simulink model "mech_stewart_control"  (Simulink 6.0)
settings: Solver=ode45  StartTime=0.0  StopTime=10.0  RelTol=1e-3
PreLoadFcn:
  | mech_stewart_control_setup
PostLoadFcn:
  | find_system(gcs,'FollowLinks', 'on', 'LookUnderMasks', 'all');set_param(gcs,'SimulationCommand','update');
undefined symbols (not defined in the file or in its folder): body_pts, pos_base, top_inertia, top_mass
libraries: simulink x10, mblibv1 x9, mech_stewartplatform_leg x6, mech_stewart_controllers x1, mech_stewart_control_deriv x1
Description:
  | Stewart platform controls case study: complete control system with
  | controller and plant.
  | 
  | Controller is one of the enabled subsystems of:
  | toolbox/physmod/mech/mechdemos/mech_stewart_controllers.mdl.
  | 
  | Plant subsystem uses leg instances of the linked library:
  | toolbox/physmod/mech/mechdemos/mech_stewartplatform_leg.mdl.
settings Model: Creator=dkennedy  LastModifiedBy=batserve  ExtModeAutoUpdateStatusClock=off
settings DataIOCC: SignalLoggingName=sigsOut  OutputTimes=[0:0.01:50]
settings OptimizationCC: BooleanDataType=off
settings DebuggingCC: CheckExecutionContextPreStartOutputMsg=on  CheckExecutionContextRuntimeOutputMsg=on  SolverPrmCheckMsg=none
settings HardwareCC: TargetUnknown=on
settings CodeAppCC: MangleLength=5
settings SimMechanicsCC: VisOnUpdateDiagram=on  VisDuringSimulation=on

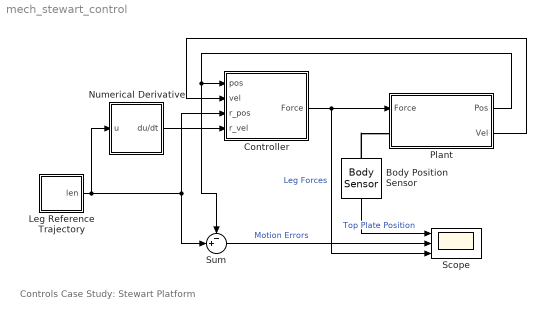
== system mech_stewart_control ==
  note: Controls Case Study:
      | Stewart Platform
  Body Position Sensor : mblibv1/Sensors &  Actuators/Body Sensor  Orientation=down  Opaque=on  PhysicalDomain=Mechanical  PortType=blob  Muxed=on  Pose=off  Angle=on  AngleUnits=deg  ArcVelocity=off  ArcVelocityUnits=deg/s  ArcAcceleration=off  ArcAccelerationUnits=deg/s^2  CoordPosition=on  CoordPositionUnits=m  Velocity=off  VelocityUnits=m/s  Acceleration=off  AccelerationUnits=m/s^2  Quaternion=on  QuaternionDT=off  QuaternionDDT=off  QuaternionUnits=off  OutputVector=[ 3 ]  ActiveIO=on  Width=3  DialogClass=MechanicalSensorBlock  ReferenceFrame=Absolute (World)
  "Controller " : Subsystem  BlockChoice=Null Controller
      settings: AttributesFormatString=%<BlockChoice>  TemplateBlock=mech_stewart_controllers/Controller  MemberBlocks=H_inf Controller,Null Controller,PID Controller
  Leg Reference Trajectory : Subsystem
  "Numerical Derivative " : Subsystem  BlockChoice=Derivative Block
      settings: AttributesFormatString=%<BlockChoice>  MemberBlocks=Derivative Block,Filtered Derivative
      settings: TemplateBlock=|
      | mech_stewart_control_deriv/Numerical
      | Derivative
  Plant : Subsystem
  Scope : Scope  NumInputPorts=3
      settings: Tag=OpenMeAtStartUp  TimeRange=1  YMin=-3~-1~-1  YMax=2~3~1
  Sum : Sum  Inputs=-+|  SaturateOnIntegerOverflow=on  InputSameDT=on
  wires:
  Plant/1(Pos) -> Sum/1, "Controller "/1(pos)
  "Controller "/1(Force) -> Plant/1(Force), Scope/3  "Leg Forces"
  Sum/1 -> Scope/2  "Motion Errors"
  Leg Reference Trajectory/1(len) -> "Numerical Derivative "/1(u), Sum/2, "Controller "/3(r_pos)
  Body Position Sensor/1 -> Scope/1  "Top Plate Position"
  Plant/2(Vel) -> "Controller "/2(vel)
  "Numerical Derivative "/1(du/dt) -> "Controller "/4(r_vel)
  connections:
  Body Position Sensor/LConn1 -- Plant/LConn1

== system mech_stewart_control/Controller  ==
  pos : Inport  Port=1  LatchInput=off
  vel : Inport  Port=2  LatchInput=off
  r_pos : Inport  Port=3  LatchInput=off
  r_vel : Inport  Port=4  LatchInput=off
  Null Controller : mech_stewart_controllers/Null Controller
  Force : Outport
  wires:
  pos/1 -> Null Controller/1
  vel/1 -> Null Controller/2
  r_pos/1 -> Null Controller/3
  r_vel/1 -> Null Controller/4
  Null Controller/1 -> Force/1

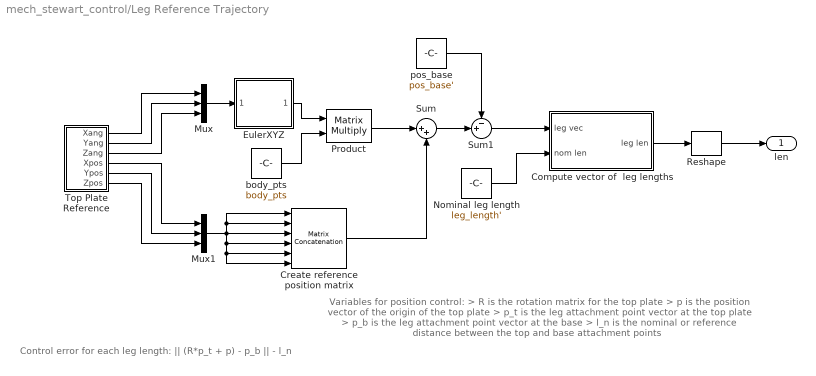
== system mech_stewart_control/Leg Reference Trajectory ==
  note: Variables for position control:
      |
      | > R is the rotation matrix  for the top plate
      | > p is the position vector of the origin of the top plate
      | > p_t is the leg attachment point vector at the top plate
      | > p_b is the leg attachment point vector at the base
      | > l_n is the nominal or reference distance between the
      |    top and base attachment points
  note: Control error for each leg length:
      |
      |    || (R*p_t + p) - p_b || - l_n
  Compute vector of  leg lengths : Subsystem  TreatAsAtomicUnit=on
  Create reference position matrix : simulink/Math Operations/Matrix Concatenation  numInports=6  catMethod=Horizontal
  EulerXYZ : Subsystem  AncestorBlock=|
      | aerospace/Axes
      | Transformations/Direction Cosine Matrix
      | from Euler Angles
      mask Type: EulerXYZ
      mask Description: Creates the EulerXYZ rotation matrix corresponding to body fixed rotations in the X, Y, and then Z. This matrix maps body vectors to world vectors.
      mask Help:
      | <p>This block determines the EulerXYZ matrix from a 3x1 euler angles in the X, Y, & Z directions. The matrix maps vectors the body axes to the inertial axes.</p>
      | 
      | <p>The block input and output contain more than one signal as described below.</p>
      | 
      | <p><H4>Block Vector Input - Euler XYZ angles</H4>
      |     <ul>
      |     <li>X angle</li>
      |     <li>Y angle</li>
      |     <li>Z angle</li>
      |    </ul>
      |    </p>
      | 
      | <p><H4>Block Matrix Output - XYZ Euler Matrix </H4>
      |     <ul>
      |    </ul>
      |    </p>
      mask Display: disp('Rotation\nMatrix')
  Mux : Mux  Inputs=3
  Mux1 : Mux  Inputs=3
  Nominal leg length : Constant  Value=leg_length'  VectorParams1D=off
  Product : Product  Multiplication=Matrix(*)  SaturateOnIntegerOverflow=on  InputSameDT=on
  Reshape : simulink/Math Operations/Reshape  OutputDimensionality=1-D array  OutputDimensions=[1,1]
  Sum : Sum  Inputs=|++  SaturateOnIntegerOverflow=on  InputSameDT=on
  Sum1 : Sum  Inputs=-+|  SaturateOnIntegerOverflow=on  InputSameDT=on
  Top Plate Reference : Subsystem
  body_pts : Constant  Value=body_pts  VectorParams1D=off
  pos_base : Constant  Value=pos_base'  VectorParams1D=off
  len : Outport
  wires:
  Mux/1 -> EulerXYZ/1(x y z angles)
  EulerXYZ/1(EulerXYZ) -> Product/1
  body_pts/1 -> Product/2
  Product/1 -> Sum/1
  Mux1/1 -> Create reference position matrix/3, Create reference position matrix/1, Create reference position matrix/2, Create reference position matrix/4, Create reference position matrix/5, Create reference position matrix/6
  Create reference position matrix/1 -> Sum/2
  pos_base/1 -> Sum1/1
  Sum/1 -> Sum1/2
  Sum1/1 -> Compute vector of  leg lengths/1(leg vec)
  Nominal leg length/1 -> Compute vector of  leg lengths/2(nom len)
  Compute vector of  leg lengths/1(leg len) -> Reshape/1
  Top Plate Reference/3(Zang) -> Mux/3
  Top Plate Reference/1(Xang) -> Mux/1
  Top Plate Reference/2(Yang) -> Mux/2
  Top Plate Reference/4(Xpos) -> Mux1/1
  Top Plate Reference/5(Ypos) -> Mux1/2
  Top Plate Reference/6(Zpos) -> Mux1/3
  Reshape/1 -> len/1

== system mech_stewart_control/Numerical Derivative  ==
  u : Inport  Port=1  LatchInput=off
  Derivative Block : mech_stewart_control_deriv/Derivative Block
  du/dt : Outport
  wires:
  u/1 -> Derivative Block/1
  Derivative Block/1 -> du/dt/1

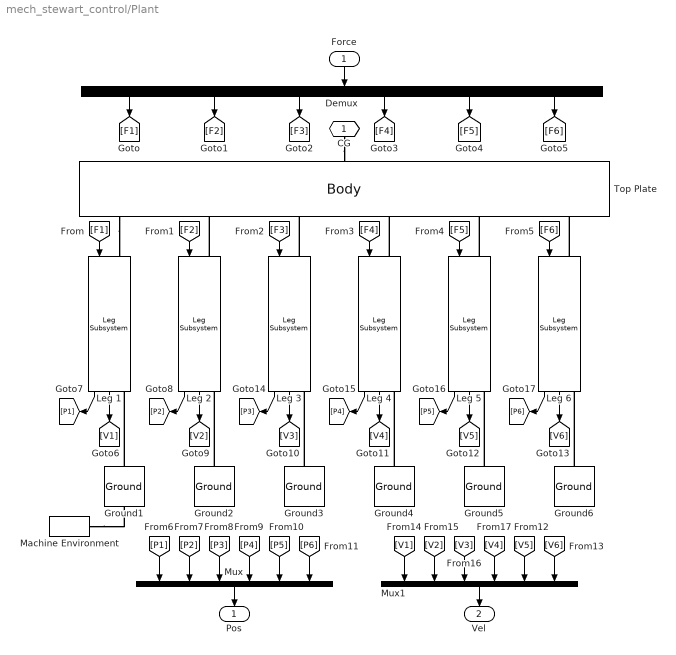
== system mech_stewart_control/Plant ==
  Force : Inport  Orientation=down  Port=1  LatchInput=off
  Demux : Demux  Orientation=down  Outputs=6
  Ground1 : mblibv1/Bodies/Ground  Orientation=up  Opaque=on  LeftPortType=env  RightPortType=workingframe  PhysicalDomain=Mechanical  DialogClass=GroundBlock  CoordPosition=pos_base(1,:)  CoordPositionUnits=m  StateVectorMgrId=-1  MachineId=[1 0]  ShowEnvPort=on
  Ground2 : mblibv1/Bodies/Ground  Orientation=up  Opaque=on  LeftPortType=env  RightPortType=workingframe  PhysicalDomain=Mechanical  DialogClass=GroundBlock  CoordPosition=pos_base(2,:)  CoordPositionUnits=m  StateVectorMgrId=-1  MachineId=[0 0]  ShowEnvPort=off
  Ground3 : mblibv1/Bodies/Ground  Orientation=up  Opaque=on  LeftPortType=env  RightPortType=workingframe  PhysicalDomain=Mechanical  DialogClass=GroundBlock  CoordPosition=pos_base(3,:)  CoordPositionUnits=m  StateVectorMgrId=-1  MachineId=[0 0]  ShowEnvPort=off
  Ground4 : mblibv1/Bodies/Ground  Orientation=up  Opaque=on  LeftPortType=env  RightPortType=workingframe  PhysicalDomain=Mechanical  DialogClass=GroundBlock  CoordPosition=pos_base(4,:)  CoordPositionUnits=m  StateVectorMgrId=-1  MachineId=[0 0]  ShowEnvPort=off
  Ground5 : mblibv1/Bodies/Ground  Orientation=up  Opaque=on  LeftPortType=env  RightPortType=workingframe  PhysicalDomain=Mechanical  DialogClass=GroundBlock  CoordPosition=pos_base(5,:)  CoordPositionUnits=m  StateVectorMgrId=-1  MachineId=[0 0]  ShowEnvPort=off
  Ground6 : mblibv1/Bodies/Ground  Orientation=up  Opaque=on  LeftPortType=env  RightPortType=workingframe  PhysicalDomain=Mechanical  DialogClass=GroundBlock  CoordPosition=pos_base(6,:)  CoordPositionUnits=m  StateVectorMgrId=-1  MachineId=[0 0]  ShowEnvPort=off
  Leg 1 : mech_stewartplatform_leg/Leg Subsystem  Orientation=down  ln=1
  Leg 2 : mech_stewartplatform_leg/Leg Subsystem  Orientation=down  ln=2
  Leg 3 : mech_stewartplatform_leg/Leg Subsystem  Orientation=down  ln=3
  Leg 4 : mech_stewartplatform_leg/Leg Subsystem  Orientation=down  ln=4
  Leg 5 : mech_stewartplatform_leg/Leg Subsystem  Orientation=down  ln=5
  Leg 6 : mech_stewartplatform_leg/Leg Subsystem  Orientation=down  ln=6
  Machine Environment : mblibv1/Bodies/Machine Environment  Tag=Factory ground  DialogController=MECH.DialogSource  Opaque=on  PortType=env  PhysicalDomain=Mechanical  DialogTemplateClass=MECH.MachineEnvironment  SyncWhenCopied=off  Gravity=[0 0 -9.81]  GravityUnits=m/s^2  GravityAsSignal=off  Dimensionality=3D Only  AnalysisType=Forward dynamics  LinearAssemblyTolerance=1e-3  LinearAssemblyToleranceUnits=m  AngularAssemblyTolerance=1e-3  AngularAssemblyToleranceUnits=rad  ConstraintSolverType=Machine precision  ConstraintRelTolerance=1e-4  ConstraintAbsTolerance=1e-4  UseRobustSingularityHandling=on  StatePerturbationType=Adaptive  PerturbationSize=1e-3  VisualizeMachine=on
  Mux : Mux  Orientation=down  Inputs=6
  Mux1 : Mux  Orientation=down  Inputs=6
  Top Plate : mblibv1/Bodies/Body  Orientation=down  PhysicalDomain=mechanical  SubClassName=Unknown  LeftPortType=workingframe  RightPortType=workingframe  LConnTagsString=CG  RConnTagsString=CS1|CS2|CS3|CS4|CS5|CS6  DialogClass=MechanicalBodyBlock  Mass=top_mass  MassUnits=kg  InertiaUnits=kg*m^2  Inertia=top_inertia  Shape=Cylinder  ShapeDims=[1 1]  ShapeUnits=m  ShapeUse=false  Density=1  DensityUnits=kg/m^3  DensityUse=false  CG=Left$CG$[0 0 height]$WORLD$WORLD$m$[0 0 0]$Euler X-Y-Z$deg$WORLD$true  WorkingFrames=Right$CS1$pos_top(1,:)$WORLD$WORLD$m$[0 0 0]$Euler X-Y-Z$deg$WORLD$true#Right$CS2$pos_top(2,:)$WORLD$WORLD$m$[0 0 0]$Euler X-Y-Z$deg$WORLD$true#Right$CS3$pos_top(3,:)$WORLD$WORLD$m$[0 0 0]$Euler X-Y-Z$deg$WORLD$true#Right$CS4$pos_top(4,:)$WORLD$WORLD$m$[0 0 0]$Euler X-Y-Z$deg$WORLD$true#Right$CS5$pos_top(5,:)$WORLD$WORLD$m$[0 0 0]$Euler X-Y-Z$deg$WORLD$true#Right$CS6$pos_top(6,:)$WORLD$WORLD$m$[0 0 0]$Euler X-Y-Z$deg$WORLD$true
  CG : PMIOPort  Orientation=down  Port=1  Side=Left
  Pos : Outport  Orientation=down
  Vel : Outport  Orientation=down  Port=2
  wires:
  Force/1 -> Demux/1
  Mux/1 -> Pos/1
  Demux/1 -> [F1]
  Demux/2 -> [F2]
  Demux/3 -> [F3]
  Demux/4 -> [F4]
  Demux/5 -> [F5]
  Demux/6 -> [F6]
  [F1] -> Leg 1/1
  [F2] -> Leg 2/1
  [F3] -> Leg 3/1
  [F4] -> Leg 4/1
  [F5] -> Leg 5/1
  [F6] -> Leg 6/1
  Leg 1/2 -> [V1]
  Leg 1/1 -> [P1]
  Leg 2/2 -> [V2]
  Leg 3/2 -> [V3]
  Leg 4/2 -> [V4]
  Leg 5/2 -> [V5]
  Leg 6/2 -> [V6]
  Leg 2/1 -> [P2]
  Leg 3/1 -> [P3]
  Leg 4/1 -> [P4]
  Leg 5/1 -> [P5]
  Leg 6/1 -> [P6]
  [P1] -> Mux/1
  [P2] -> Mux/2
  [P3] -> Mux/3
  [P4] -> Mux/4
  [P5] -> Mux/5
  [P6] -> Mux/6
  [V1] -> Mux1/1
  [V2] -> Mux1/2
  [V3] -> Mux1/3
  [V4] -> Mux1/4
  [V5] -> Mux1/5
  [V6] -> Mux1/6
  Mux1/1 -> Vel/1
  connections:
  Top Plate/RConn1 -- Leg 1/LConn1
  Ground6/RConn1 -- Leg 6/RConn1
  Ground5/RConn1 -- Leg 5/RConn1
  Ground4/RConn1 -- Leg 4/RConn1
  Ground3/RConn1 -- Leg 3/RConn1
  Ground2/RConn1 -- Leg 2/RConn1
  Ground1/RConn1 -- Leg 1/RConn1
  Leg 2/LConn1 -- Top Plate/RConn2
  Leg 3/LConn1 -- Top Plate/RConn3
  Leg 4/LConn1 -- Top Plate/RConn4
  Leg 5/LConn1 -- Top Plate/RConn5
  Leg 6/LConn1 -- Top Plate/RConn6
  CG/RConn1 -- Top Plate/LConn1
  Machine Environment/RConn1 -- Ground1/LConn1

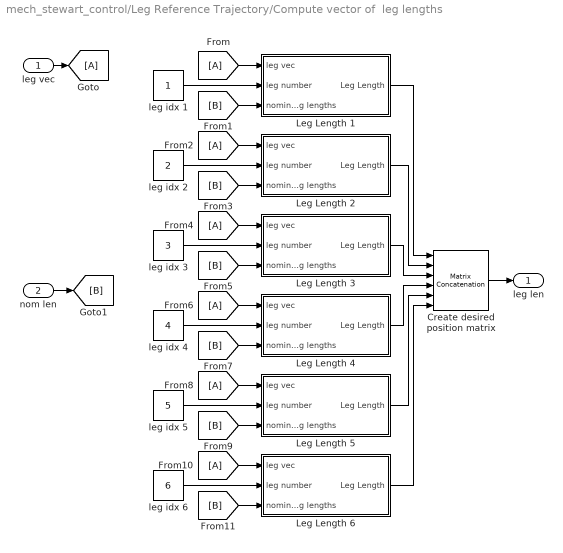
== system mech_stewart_control/Leg Reference Trajectory/Compute vector of  leg lengths ==
  leg vec : Inport  Port=1  LatchInput=off
  nom len : Inport  Port=2  LatchInput=off
  Create desired position matrix : simulink/Math Operations/Matrix Concatenation  numInports=6  catMethod=Horizontal
  Leg Length 1 : Subsystem
  Leg Length 2 : Subsystem
  Leg Length 3 : Subsystem
  Leg Length 4 : Subsystem
  Leg Length 5 : Subsystem
  Leg Length 6 : Subsystem
  leg idx 1 : Constant
  leg idx 2 : Constant  Value=2
  leg idx 3 : Constant  Value=3
  leg idx 4 : Constant  Value=4
  leg idx 5 : Constant  Value=5
  leg idx 6 : Constant  Value=6
  leg len : Outport
  wires:
  Leg Length 6/1(Leg Length) -> Create desired position matrix/6
  Leg Length 5/1(Leg Length) -> Create desired position matrix/5
  Leg Length 4/1(Leg Length) -> Create desired position matrix/4
  Leg Length 3/1(Leg Length) -> Create desired position matrix/3
  Leg Length 2/1(Leg Length) -> Create desired position matrix/2
  Leg Length 1/1(Leg Length) -> Create desired position matrix/1
  [B] -> Leg Length 6/3(nominal leg lengths)
  [A] -> Leg Length 6/1(leg vec)
  leg idx 6/1 -> Leg Length 6/2(leg number)
  [B] -> Leg Length 5/3(nominal leg lengths)
  [A] -> Leg Length 5/1(leg vec)
  leg idx 5/1 -> Leg Length 5/2(leg number)
  [B] -> Leg Length 4/3(nominal leg lengths)
  [A] -> Leg Length 4/1(leg vec)
  leg idx 4/1 -> Leg Length 4/2(leg number)
  [B] -> Leg Length 3/3(nominal leg lengths)
  [A] -> Leg Length 3/1(leg vec)
  leg idx 3/1 -> Leg Length 3/2(leg number)
  [B] -> Leg Length 2/3(nominal leg lengths)
  [A] -> Leg Length 2/1(leg vec)
  leg idx 2/1 -> Leg Length 2/2(leg number)
  [B] -> Leg Length 1/3(nominal leg lengths)
  nom len/1 -> [B]
  [A] -> Leg Length 1/1(leg vec)
  leg vec/1 -> [A]
  leg idx 1/1 -> Leg Length 1/2(leg number)
  Create desired position matrix/1 -> leg len/1

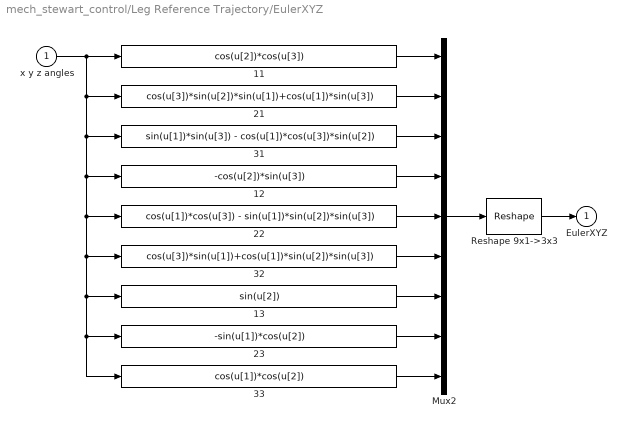
== system mech_stewart_control/Leg Reference Trajectory/EulerXYZ ==
  x y z angles : Inport  Port=1  LatchInput=off
  11 : Fcn  Expr=cos(u[2])*cos(u[3])
  12 : Fcn  Expr=-cos(u[2])*sin(u[3])
  13 : Fcn  Expr=sin(u[2])
  21 : Fcn  Expr=cos(u[3])*sin(u[2])*sin(u[1])+cos(u[1])*sin(u[3])
  22 : Fcn  Expr=cos(u[1])*cos(u[3]) - sin(u[1])*sin(u[2])*sin(u[3])
  23 : Fcn  Expr=-sin(u[1])*cos(u[2])
  31 : Fcn  Expr=sin(u[1])*sin(u[3]) - cos(u[1])*cos(u[3])*sin(u[2])
  32 : Fcn  Expr=cos(u[3])*sin(u[1])+cos(u[1])*sin(u[2])*sin(u[3])
  33 : Fcn  Expr=cos(u[1])*cos(u[2])
  Mux2 : Mux  Inputs=9
  Reshape 9x1->3x3 : simulink/Math Operations/Reshape  OutputDimensionality=Customize  OutputDimensions=[3,3]
  EulerXYZ : Outport  InitialOutput=0
  wires:
  x y z angles/1 -> 23/1, 33/1, 13/1, 32/1, 22/1, 12/1, 31/1, 21/1, 11/1
  33/1 -> Mux2/9
  23/1 -> Mux2/8
  13/1 -> Mux2/7
  32/1 -> Mux2/6
  22/1 -> Mux2/5
  12/1 -> Mux2/4
  31/1 -> Mux2/3
  21/1 -> Mux2/2
  11/1 -> Mux2/1
  Mux2/1 -> Reshape 9x1->3x3/1
  Reshape 9x1->3x3/1 -> EulerXYZ/1

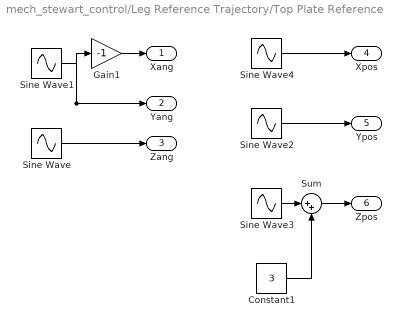
== system mech_stewart_control/Leg Reference Trajectory/Top Plate Reference ==
  Constant1 : Constant  Value=3
  Gain1 : Gain  Gain=-1  SaturateOnIntegerOverflow=on
  Sine Wave : Sin  Amplitude=0.3  Frequency=3  SampleTime=0
  Sine Wave1 : Sin  Amplitude=0.3  Frequency=3  SampleTime=0
  Sine Wave2 : Sin  Amplitude=0.25  Frequency=3  Phase=pi/2  SampleTime=0
  Sine Wave3 : Sin  Amplitude=0.25  Frequency=3  SampleTime=0
  Sine Wave4 : Sin  Amplitude=0.5  Frequency=3  SampleTime=0
  Sum : Sum  Inputs=|++  SaturateOnIntegerOverflow=on  InputSameDT=on
  Xang : Outport
  Yang : Outport  Port=2
  Zang : Outport  Port=3
  Xpos : Outport  Port=4
  Ypos : Outport  Port=5
  Zpos : Outport  Port=6
  wires:
  Sine Wave/1 -> Zang/1
  Sine Wave1/1 -> Gain1/1, Yang/1
  Gain1/1 -> Xang/1
  Sine Wave2/1 -> Ypos/1
  Sine Wave3/1 -> Sum/1
  Sum/1 -> Zpos/1
  Constant1/1 -> Sum/2
  Sine Wave4/1 -> Xpos/1

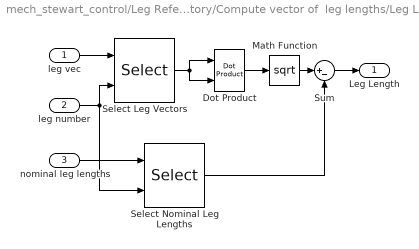
== system mech_stewart_control/Leg Reference Trajectory/Compute vector of  leg lengths/Leg Length 1 ==
  leg vec : Inport  Port=1  LatchInput=off
  leg number : Inport  Port=2  LatchInput=off
  nominal leg lengths : Inport  Port=3  LatchInput=off
  Dot Product : simulink/Math Operations/Dot Product  OutDataType=sfix(16)  OutScaling=2^-10  DoSatur=off
  Math Function : Math  Operator=sqrt  SaturateOnIntegerOverflow=on
  Select Leg Vectors : Selector  InputType=Matrix  ElementSrc=External  Elements=[1 3]  Rows=-1  ColumnSrc=External  InputPortWidth=3
  Select Nominal Leg Lengths : Selector  ElementSrc=External  Elements=[1 3]  Rows=-1  ColumnSrc=External  InputPortWidth=6
  Sum : Sum  Inputs=|+-  SaturateOnIntegerOverflow=on  InputSameDT=on
  Leg Length : Outport
  wires:
  nominal leg lengths/1 -> Select Nominal Leg Lengths/1
  Sum/1 -> Leg Length/1
  leg vec/1 -> Select Leg Vectors/1
  leg number/1 -> Select Leg Vectors/2, Select Nominal Leg Lengths/2
  Dot Product/1 -> Math Function/1
  Select Leg Vectors/1 -> Dot Product/1, Dot Product/2
  Math Function/1 -> Sum/1
  Select Nominal Leg Lengths/1 -> Sum/2

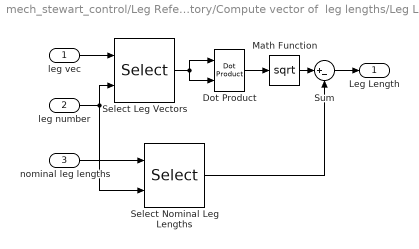
== system mech_stewart_control/Leg Reference Trajectory/Compute vector of  leg lengths/Leg Length 2 ==
  leg vec : Inport  Port=1  LatchInput=off
  leg number : Inport  Port=2  LatchInput=off
  nominal leg lengths : Inport  Port=3  LatchInput=off
  Dot Product : simulink/Math Operations/Dot Product  OutDataType=sfix(16)  OutScaling=2^-10  DoSatur=off
  Math Function : Math  Operator=sqrt  SaturateOnIntegerOverflow=on
  Select Leg Vectors : Selector  InputType=Matrix  ElementSrc=External  Elements=[1 3]  Rows=-1  ColumnSrc=External  InputPortWidth=3
  Select Nominal Leg Lengths : Selector  ElementSrc=External  Elements=[1 3]  Rows=-1  ColumnSrc=External  InputPortWidth=6
  Sum : Sum  Inputs=|+-  SaturateOnIntegerOverflow=on  InputSameDT=on
  Leg Length : Outport
  wires:
  nominal leg lengths/1 -> Select Nominal Leg Lengths/1
  Sum/1 -> Leg Length/1
  leg vec/1 -> Select Leg Vectors/1
  leg number/1 -> Select Leg Vectors/2, Select Nominal Leg Lengths/2
  Dot Product/1 -> Math Function/1
  Select Leg Vectors/1 -> Dot Product/1, Dot Product/2
  Math Function/1 -> Sum/1
  Select Nominal Leg Lengths/1 -> Sum/2

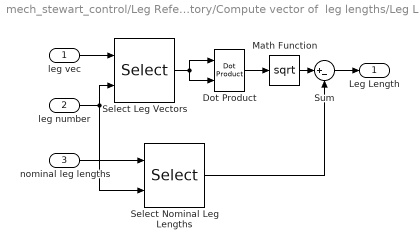
== system mech_stewart_control/Leg Reference Trajectory/Compute vector of  leg lengths/Leg Length 3 ==
  leg vec : Inport  Port=1  LatchInput=off
  leg number : Inport  Port=2  LatchInput=off
  nominal leg lengths : Inport  Port=3  LatchInput=off
  Dot Product : simulink/Math Operations/Dot Product  OutDataType=sfix(16)  OutScaling=2^-10  DoSatur=off
  Math Function : Math  Operator=sqrt  SaturateOnIntegerOverflow=on
  Select Leg Vectors : Selector  InputType=Matrix  ElementSrc=External  Elements=[1 3]  Rows=-1  ColumnSrc=External  InputPortWidth=3
  Select Nominal Leg Lengths : Selector  ElementSrc=External  Elements=[1 3]  Rows=-1  ColumnSrc=External  InputPortWidth=6
  Sum : Sum  Inputs=|+-  SaturateOnIntegerOverflow=on  InputSameDT=on
  Leg Length : Outport
  wires:
  nominal leg lengths/1 -> Select Nominal Leg Lengths/1
  Sum/1 -> Leg Length/1
  leg vec/1 -> Select Leg Vectors/1
  leg number/1 -> Select Leg Vectors/2, Select Nominal Leg Lengths/2
  Dot Product/1 -> Math Function/1
  Select Leg Vectors/1 -> Dot Product/1, Dot Product/2
  Math Function/1 -> Sum/1
  Select Nominal Leg Lengths/1 -> Sum/2

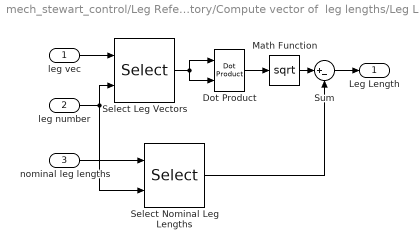
== system mech_stewart_control/Leg Reference Trajectory/Compute vector of  leg lengths/Leg Length 4 ==
  leg vec : Inport  Port=1  LatchInput=off
  leg number : Inport  Port=2  LatchInput=off
  nominal leg lengths : Inport  Port=3  LatchInput=off
  Dot Product : simulink/Math Operations/Dot Product  OutDataType=sfix(16)  OutScaling=2^-10  DoSatur=off
  Math Function : Math  Operator=sqrt  SaturateOnIntegerOverflow=on
  Select Leg Vectors : Selector  InputType=Matrix  ElementSrc=External  Elements=[1 3]  Rows=-1  ColumnSrc=External  InputPortWidth=3
  Select Nominal Leg Lengths : Selector  ElementSrc=External  Elements=[1 3]  Rows=-1  ColumnSrc=External  InputPortWidth=6
  Sum : Sum  Inputs=|+-  SaturateOnIntegerOverflow=on  InputSameDT=on
  Leg Length : Outport
  wires:
  nominal leg lengths/1 -> Select Nominal Leg Lengths/1
  Sum/1 -> Leg Length/1
  leg vec/1 -> Select Leg Vectors/1
  leg number/1 -> Select Leg Vectors/2, Select Nominal Leg Lengths/2
  Dot Product/1 -> Math Function/1
  Select Leg Vectors/1 -> Dot Product/1, Dot Product/2
  Math Function/1 -> Sum/1
  Select Nominal Leg Lengths/1 -> Sum/2

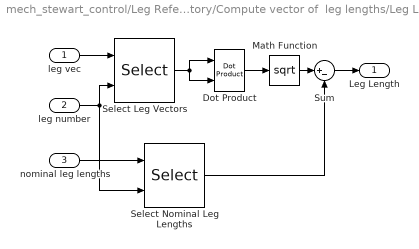
== system mech_stewart_control/Leg Reference Trajectory/Compute vector of  leg lengths/Leg Length 5 ==
  leg vec : Inport  Port=1  LatchInput=off
  leg number : Inport  Port=2  LatchInput=off
  nominal leg lengths : Inport  Port=3  LatchInput=off
  Dot Product : simulink/Math Operations/Dot Product  OutDataType=sfix(16)  OutScaling=2^-10  DoSatur=off
  Math Function : Math  Operator=sqrt  SaturateOnIntegerOverflow=on
  Select Leg Vectors : Selector  InputType=Matrix  ElementSrc=External  Elements=[1 3]  Rows=-1  ColumnSrc=External  InputPortWidth=3
  Select Nominal Leg Lengths : Selector  ElementSrc=External  Elements=[1 3]  Rows=-1  ColumnSrc=External  InputPortWidth=6
  Sum : Sum  Inputs=|+-  SaturateOnIntegerOverflow=on  InputSameDT=on
  Leg Length : Outport
  wires:
  nominal leg lengths/1 -> Select Nominal Leg Lengths/1
  Sum/1 -> Leg Length/1
  leg vec/1 -> Select Leg Vectors/1
  leg number/1 -> Select Leg Vectors/2, Select Nominal Leg Lengths/2
  Dot Product/1 -> Math Function/1
  Select Leg Vectors/1 -> Dot Product/1, Dot Product/2
  Math Function/1 -> Sum/1
  Select Nominal Leg Lengths/1 -> Sum/2

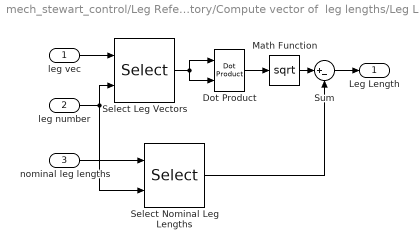
== system mech_stewart_control/Leg Reference Trajectory/Compute vector of  leg lengths/Leg Length 6 ==
  leg vec : Inport  Port=1  LatchInput=off
  leg number : Inport  Port=2  LatchInput=off
  nominal leg lengths : Inport  Port=3  LatchInput=off
  Dot Product : simulink/Math Operations/Dot Product  OutDataType=sfix(16)  OutScaling=2^-10  DoSatur=off
  Math Function : Math  Operator=sqrt  SaturateOnIntegerOverflow=on
  Select Leg Vectors : Selector  InputType=Matrix  ElementSrc=External  Elements=[1 3]  Rows=-1  ColumnSrc=External  InputPortWidth=3
  Select Nominal Leg Lengths : Selector  ElementSrc=External  Elements=[1 3]  Rows=-1  ColumnSrc=External  InputPortWidth=6
  Sum : Sum  Inputs=|+-  SaturateOnIntegerOverflow=on  InputSameDT=on
  Leg Length : Outport
  wires:
  nominal leg lengths/1 -> Select Nominal Leg Lengths/1
  Sum/1 -> Leg Length/1
  leg vec/1 -> Select Leg Vectors/1
  leg number/1 -> Select Leg Vectors/2, Select Nominal Leg Lengths/2
  Dot Product/1 -> Math Function/1
  Select Leg Vectors/1 -> Dot Product/1, Dot Product/2
  Math Function/1 -> Sum/1
  Select Nominal Leg Lengths/1 -> Sum/2
